simulink model "input_signal"  (Simulink 7.4)
settings: Solver=VariableStepDiscrete  StartTime=0.0  StopTime=10.0  MaxStep=0.0001  RelTol=1e-3
settings Model: Creator=Vittorio  LastModifiedBy=Vittorio

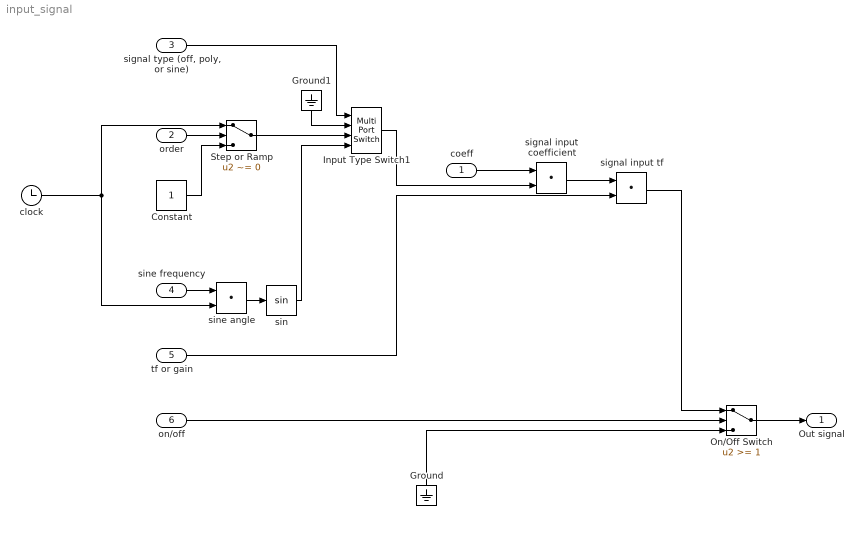
== system input_signal ==
  coeff : Inport  OutDataType=fixdt(1, 16)  OutScaling=2^0
  order : Inport  Port=2  OutDataType=fixdt(1, 16)  OutScaling=2^0
  "signal type (off, poly, or sine)" : Inport  Port=3  OutDataType=fixdt(1, 16)  OutScaling=2^0
  sine frequency : Inport  Port=4  OutDataType=fixdt(1, 16)  OutScaling=2^0
  tf or gain : Inport  Port=5  OutDataType=fixdt(1, 16)  OutScaling=2^0
  on/off : Inport  Port=6  OutDataType=fixdt(1, 16)  OutScaling=2^0
  Constant : Constant  OutDataType=fixdt(1, 16)  OutScaling=2^0
  Ground : Ground
  Ground1 : Ground
  Input Type Switch1 : MultiPortSwitch  zeroidx=on  OutDataType=fixdt(1, 16)  OutScaling=2^0
  On/Off Switch : Switch  Threshold=1
  Step or Ramp : Switch  Criteria=u2 ~= 0  Threshold=1
  clock : Clock
      settings: Decimation=10
  signal input coefficient : DotProduct  OutDataType=fixdt(1, 16)  OutScaling=2^-10  InputSameDT=on  OutDataTypeStr=Inherit: Inherit via internal rule
  signal input tf : DotProduct  OutDataType=fixdt(1, 16)  OutScaling=2^-10  InputSameDT=on  OutDataTypeStr=Inherit: Inherit via internal rule
  sin : Trigonometry
  sine angle : DotProduct  OutDataType=fixdt(1, 16)  OutScaling=2^-10  InputSameDT=on  OutDataTypeStr=Inherit: Inherit via internal rule
  Out signal : Outport  OutDataType=fixdt(1, 16)  OutScaling=2^0
  wires:
  Ground/1 -> On/Off Switch/3
  on/off/1 -> On/Off Switch/2
  On/Off Switch/1 -> Out signal/1
  sine angle/1 -> sin/1
  sine frequency/1 -> sine angle/1
  sin/1 -> Input Type Switch1/4
  order/1 -> Step or Ramp/2
  coeff/1 -> signal input coefficient/1
  Input Type Switch1/1 -> signal input coefficient/2
  "signal type (off, poly, or sine)"/1 -> Input Type Switch1/1
  Ground1/1 -> Input Type Switch1/2
  Step or Ramp/1 -> Input Type Switch1/3
  signal input coefficient/1 -> signal input tf/1
  tf or gain/1 -> signal input tf/2
  signal input tf/1 -> On/Off Switch/1
  clock/1 -> sine angle/2, Step or Ramp/1
  Constant/1 -> Step or Ramp/3
